simulink model "kaskadka2"  (R2013a)
settings: Solver=ode45  StartTime=0.0  StopTime=20.0  RelTol=1e-3  AbsTol=1e-6
values from neighbouring files (symbols this model uses):
  A1 = 1    [Kaskady.m]    (also in Kaskady2.m; Palmowski.m = -1/(1-lam1/lam2); transmitacje.m)
  A2 = 1    [Kaskady.m]    (also in Kaskady2.m; Palmowski.m = -1-A1; transmitacje.m)
  Aw1 = 0.1    [Kaskady.m]    (also in Kaskady2.m; transmitacje.m)
  Aw2 = 0.1    [Kaskady.m]    (also in Kaskady2.m; transmitacje.m)
  dfwew1 = 0.1*fwew1max    [Kaskady.m]    (also in Kaskady2.m = 0; transmitacje.m)
  dfwew2 = 0.1*fwew2max    [Kaskady.m]    (also in Kaskady2.m; transmitacje.m)
  fwew1 = k(i)*fwew1max    [Kaskady.m]    (also in Kaskady2.m = 0.1; transmitacje.m = 0)
  fwew2 = 0.1    [Kaskady.m]    (also in Kaskady2.m = k(i)*fwew2max; transmitacje.m = 0)
  g = 10    [Kaskady.m]    (also in Kaskady2.m; transmitacje.m = 9.8)
  h10 = fwew1/a1    [Kaskady.m]    (also in Kaskady2.m; transmitacje.m)
  h20 = (fwew1+fwew2)/a2    [Kaskady.m]    (also in Kaskady2.m; transmitacje.m)
  t0 = 1    [Kaskady.m]    (also in Kaskady2.m; Skoki.m = 0; symulek1.m; transmitacje.m)
settings Model: Creator=LAB320-1552  LastModifiedBy=LAB320-1552
settings DebuggingCC: SolverPrmCheckMsg=none

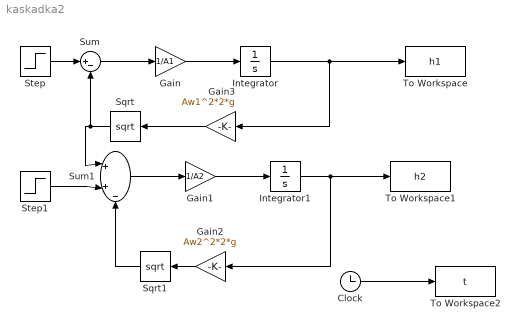
== system kaskadka2 ==
  Clock : Clock
  Gain : Gain  Gain=1/A1
  Gain1 : Gain  Gain=1/A2
  Gain2 : Gain  Gain=Aw2^2*2*g
  Gain3 : Gain  Gain=Aw1^2*2*g
  Integrator : Integrator  InitialCondition=h10
  Integrator1 : Integrator  InitialCondition=h20
  Sqrt : Sqrt  SaturateOnIntegerOverflow=on
  Sqrt1 : Sqrt  SaturateOnIntegerOverflow=on
  Step : Step  Time=t0  Before=fwew1  After=fwew1+dfwew1  SampleTime=0
  Step1 : Step  Time=t0  Before=fwew2  After=fwew2+dfwew2  SampleTime=0
  Sum : Sum  Inputs=|+-
  Sum1 : Sum  Inputs=|++-
  To Workspace : ToWorkspace  VariableName=h1  SampleTime=-1
  To Workspace1 : ToWorkspace  VariableName=h2  SampleTime=-1
  To Workspace2 : ToWorkspace  VariableName=t  SampleTime=-1  SaveFormat=Timeseries
  wires:
  Clock/1 -> To Workspace2/1
  Step/1 -> Sum/1
  Integrator/1 -> Gain3/1, To Workspace/1
  Sum/1 -> Gain/1
  Gain/1 -> Integrator/1
  Step1/1 -> Sum1/2
  Gain2/1 -> Sqrt1/1
  Sum1/1 -> Gain1/1
  Gain1/1 -> Integrator1/1
  Integrator1/1 -> Gain2/1, To Workspace1/1
  Gain3/1 -> Sqrt/1
  Sqrt/1 -> Sum1/1, Sum/2
  Sqrt1/1 -> Sum1/3
